simulink model "test_model"  (R2022b)
settings: Solver=VariableStepAuto  StartTime=0.0  StopTime=10.0  RelTol=1e-3
InitFcn:
  | parameters_test_model;
values from neighbouring files (symbols this model uses):
  A1 = [0.3, 0.3, 0.2]    [parameters_test_model.m]    (also in tensegrity_Val_like.m = [(G1+G2+G3)/3])
  a1 = 0.04    [parameters_test_model.m]
  b_all = 2*ones(6, 1)    [parameters_test_model.m]
  h1 = 0.5    [parameters_test_model.m]
  k_all = 1e3*ones(6, 1)    [parameters_test_model.m]
  l0_all = [l01, l02, l03, l04, l05, l06]'    [parameters_test_model.m]
  predpeti = 0.95    [parameters_test_model.m]
undefined symbols (not defined in the file or in its folder): X, Y, Z
libraries: sm_lib x21, nesl_utility x21
settings Model: Creator=zavrel  LastModifiedBy=zavrel
settings SolverCC: AlgebraicLoopSolver=TrustRegion
settings DebuggingCC: UnconnectedInputMsg=warning  UnconnectedOutputMsg=warning  UnconnectedLineMsg=warning  SFMachineParentedDataDiag=warning
settings ModelReferenceCC: EnableRefExpFcnMdlSchedulingChecks=on
settings RTWCC: DLArmComputeVersion=19.05

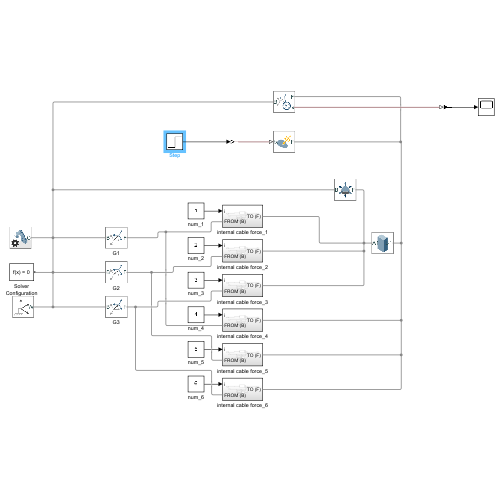
[thumbnail: Simulink's stored preview of the top-level diagram]
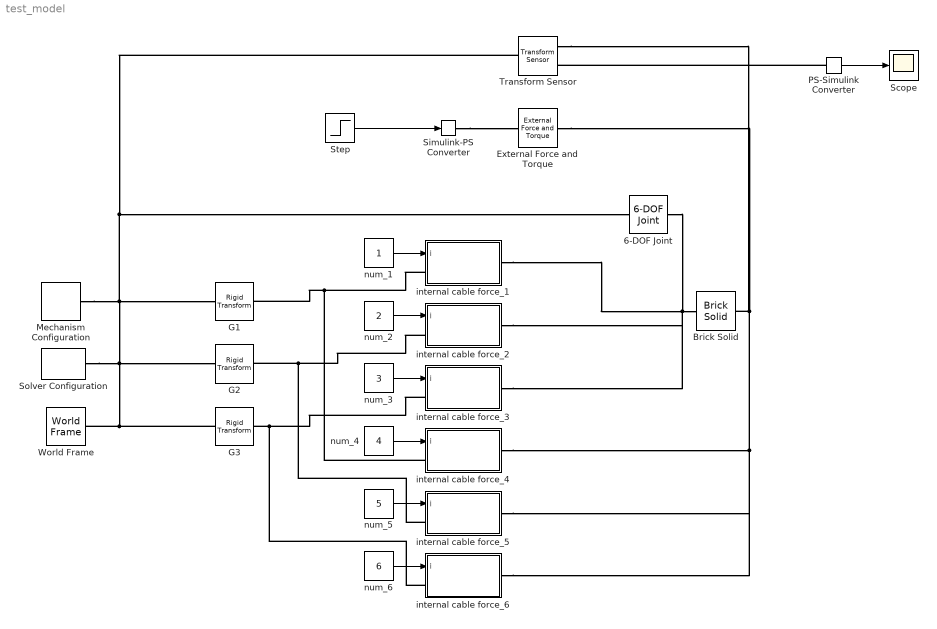
== system test_model ==
  6-DOF Joint : sm_lib/Joints/6-DOF Joint  JointMode=Normal  SenseConstraintForce=off  SenseConstraintForceX=off  SenseConstraintForceY=off  SenseConstraintForceZ=off  SenseConstraintTorque=off  SenseConstraintTorqueX=off  SenseConstraintTorqueY=off  SenseConstraintTorqueZ=off  SenseTotalForce=off  SenseTotalForceX=off  SenseTotalForceY=off  SenseTotalForceZ=off  SenseTotalTorque=off  SenseTotalTorqueX=off  SenseTotalTorqueY=off  SenseTotalTorqueZ=off  CompositeWrenchDir=FollowerOnBase  CompositeWrenchFrame=BaseFrame  PxEquilibriumPosition=0  PxEquilibriumPositionUnits=m  PxSpringStiffness=0  PxSpringStiffnessUnits=N/m  PxDampingCoefficient=0  PxDampingCoefficientUnits=N/(m/s)  PxTorqueActuationMode=NoTorque  PxMotionActuationMode=ComputedMotion  PxSensePosition=off  PxSenseVelocity=off  PxSenseAcceleration=off  PxSenseTorqueForce=off  PxSenseLowerLimitTorqueForce=off  PxSenseUpperLimitTorqueForce=off  PxLowerLimitSpecify=off  PxLowerLimitBound=-1  PxLowerLimitBoundUnits=m  PxLowerLimitStiffness=1e6  PxLowerLimitStiffnessUnits=N/m  PxLowerLimitDamping=1e3  PxLowerLimitDampingUnits=N/(m/s)  PxLowerLimitTransitionRegionWidth=1e-4  PxLowerLimitTransitionRegionWidthUnits=m  PxUpperLimitSpecify=off  PxUpperLimitBound=1  PxUpperLimitBoundUnits=m  PxUpperLimitStiffness=1e6  PxUpperLimitStiffnessUnits=N/m  PxUpperLimitDamping=1e3  PxUpperLimitDampingUnits=N/(m/s)  PxUpperLimitTransitionRegionWidth=1e-4  PxUpperLimitTransitionRegionWidthUnits=m  PxPositionTargetSpecify=on  PxPositionTargetPriority=Low  PxPositionTargetValue=A1(1)  PxPositionTargetValueUnits=m  PxVelocityTargetSpecify=off  PxVelocityTargetPriority=High  PxVelocityTargetValue=0  PxVelocityTargetValueUnits=m/s  PyEquilibriumPosition=0  PyEquilibriumPositionUnits=m  PySpringStiffness=0  PySpringStiffnessUnits=N/m  PyDampingCoefficient=0  PyDampingCoefficientUnits=N/(m/s)  PyTorqueActuationMode=NoTorque  PyMotionActuationMode=ComputedMotion  PySensePosition=off  PySenseVelocity=off  PySenseAcceleration=off  PySenseTorqueForce=off  PySenseLowerLimitTorqueForce=off  PySenseUpperLimitTorqueForce=off  PyLowerLimitSpecify=off  PyLowerLimitBound=-1  PyLowerLimitBoundUnits=m  PyLowerLimitStiffness=1e6  PyLowerLimitStiffnessUnits=N/m  PyLowerLimitDamping=1e3  PyLowerLimitDampingUnits=N/(m/s)  PyLowerLimitTransitionRegionWidth=1e-4  PyLowerLimitTransitionRegionWidthUnits=m  PyUpperLimitSpecify=off  PyUpperLimitBound=1  PyUpperLimitBoundUnits=m  PyUpperLimitStiffness=1e6  PyUpperLimitStiffnessUnits=N/m  PyUpperLimitDamping=1e3  PyUpperLimitDampingUnits=N/(m/s)  PyUpperLimitTransitionRegionWidth=1e-4  PyUpperLimitTransitionRegionWidthUnits=m  PyPositionTargetSpecify=on  PyPositionTargetPriority=Low  PyPositionTargetValue=A1(2)  PyPositionTargetValueUnits=m  PyVelocityTargetSpecify=off  PyVelocityTargetPriority=High  PyVelocityTargetValue=0  PyVelocityTargetValueUnits=m/s  PzEquilibriumPosition=0  PzEquilibriumPositionUnits=m  PzSpringStiffness=0  PzSpringStiffnessUnits=N/m  PzDampingCoefficient=0  PzDampingCoefficientUnits=N/(m/s)  PzTorqueActuationMode=NoTorque  PzMotionActuationMode=ComputedMotion  PzSensePosition=off  PzSenseVelocity=off  PzSenseAcceleration=off  PzSenseTorqueForce=off  PzSenseLowerLimitTorqueForce=off  PzSenseUpperLimitTorqueForce=off  PzLowerLimitSpecify=off  PzLowerLimitBound=-1  PzLowerLimitBoundUnits=m  PzLowerLimitStiffness=1e6  PzLowerLimitStiffnessUnits=N/m  PzLowerLimitDamping=1e3  PzLowerLimitDampingUnits=N/(m/s)  PzLowerLimitTransitionRegionWidth=1e-4  PzLowerLimitTransitionRegionWidthUnits=m  PzUpperLimitSpecify=off  PzUpperLimitBound=1  PzUpperLimitBoundUnits=m  PzUpperLimitStiffness=1e6  PzUpperLimitStiffnessUnits=N/m  PzUpperLimitDamping=1e3  PzUpperLimitDampingUnits=N/(m/s)  PzUpperLimitTransitionRegionWidth=1e-4  PzUpperLimitTransitionRegionWidthUnits=m  PzPositionTargetSpecify=on  PzPositionTargetPriority=Low  PzPositionTargetValue=A1(3)  PzPositionTargetValueUnits=m  PzVelocityTargetSpecify=off  PzVelocityTargetPriority=High  PzVelocityTargetValue=0  PzVelocityTargetValueUnits=m/s  SphEqPosRotationMethod=None  SphEqPosRotationAngleUnits=deg  SphEqPosRotationStandardAxis=+Z  SphEqPosRotationAngle=0.0  SphEqPosRotationArbitraryAxis=[0 0 1]  SphEqPosFollAlignAxisA=+X  SphEqPosBaseAlignAxisA=+Y  SphEqPosFollAlignAxisB=+Y  SphEqPosBaseAlignAxisB=+Z  SphEqPosRotationSequenceAxes=FollowerAxes  SphEqPosRotationSequence=XYX  SphEqPosRotationSequenceAngles=[0 0 0]  SphEqPosRotationSequenceAnglesUnits=deg  SphEqPosRotationMatrix=[1 0 0; 0 1 0; 0 0 1]  SphEqPosQuaternion=[1 0 0 0]  SphSpringStiffness=0  SphSpringStiffnessUnits=N*m/deg  SphDampingCoefficient=0  SphDampingCoefficientUnits=N*m/(deg/s)  SphActuateTorqueX=off  SphActuateTorqueY=off  SphActuateTorqueZ=off  SphActuateTorque=off  SphTorqueActuationMode=NoTorque  SphMotionActuationMode=ComputedMotion  SphActuationFrame=BaseFrame  SphSensePosition=off  SphSenseVelocityX=off  SphSenseVelocityY=off  SphSenseVelocityZ=off  SphSenseVelocity=off  SphSenseAccelerationX=off  SphSenseAccelerationY=off  SphSenseAccelerationZ=off  SphSenseAcceleration=off  SphSenseTorqueX=off  SphSenseTorqueY=off  SphSenseTorqueZ=off  SphSenseTorqueForce=off  SphSenseLowerLimitTorqueMag=off  SphSenseUpperLimitTorqueMag=off  SphSensingFrame=BaseFrame  SphLowerLimitSpecify=off  SphLowerLimitBound=15  SphLowerLimitBoundUnits=deg  SphLowerLimitStiffness=1e4  SphLowerLimitStiffnessUnits=N*m/deg  SphLowerLimitDamping=10  SphLowerLimitDampingUnits=N*m/(deg/s)  SphLowerLimitTransitionRegionWidth=0.1  SphLowerLimitTransitionRegionWidthUnits=deg  SphUpperLimitSpecify=off  SphUpperLimitBound=45  SphUpperLimitBoundUnits=deg  SphUpperLimitStiffness=1e4  SphUpperLimitStiffnessUnits=N*m/deg  SphUpperLimitDamping=10  SphUpperLimitDampingUnits=N*m/(deg/s)  SphUpperLimitTransitionRegionWidth=0.1  SphUpperLimitTransitionRegionWidthUnits=deg  SphPositionTargetRotationMethod=RotationSequence  SphPositionTargetRotationAngleUnits=deg  SphPositionTargetRotationStandardAxis=+Z  SphPositionTargetRotationAngle=0.0  SphPositionTargetRotationArbitraryAxis=[0 0 1]  SphPositionTargetFollAlignAxisA=+X  SphPositionTargetBaseAlignAxisA=+Y  SphPositionTargetFollAlignAxisB=+Y  SphPositionTargetBaseAlignAxisB=+Z  SphPositionTargetRotationSequenceAxes=FollowerAxes  SphPositionTargetRotationSequence=XYZ  SphPositionTargetRotationSequenceAngles=[0 0 0]  SphPositionTargetRotationSequenceAnglesUnits=deg  SphPositionTargetRotationMatrix=[1 0 0; 0 1 0; 0 0 1]  SphPositionTargetQuaternion=[1 0 0 0]  SphPositionTargetSpecify=on  SphPositionTargetPriority=Low  SphVelocityTargetValue=[0 0 0]  SphVelocityTargetValueUnits=deg/s  SphVelocityTargetSpecify=off  SphVelocityTargetPriority=High  SphVelocityTargetInFollowerFrame=on
  Brick Solid : sm_lib/Body Elements/Brick Solid  GraphicAmbientColor=[0.15 0.15 0.15 1.0]  BasedOnType=Density  BrickDimensions=[a1 a1 h1]  BrickDimensionUnits=m  CenterOfMass=[0 0 0]  CenterOfMassUnits=m  GraphicDiffuseColor=[0.5 0.5 0.5]  Density=1000  DensityUnits=kg/m^3  DoExposeReferenceFrame=off  GraphicEmissiveColor=[0.0 0.0 0.0 1.0]  ExportEntireGeometry=off  SerializedFrames=<Frames><Frame><Id>Frame1</Id><Value><Name>A1</Name><Origin><Source>GeometricFeature</Source><FeatureName>-z surface</FeatureName></Origin><PrimaryAxis><DefinedDirection>+Z</DefinedDirection><Source>ReferenceFrame</Source><SourceDirection>+Z</SourceDirection><FeatureName></FeatureName></PrimaryAxis><SecondaryAxis><DefinedDirection>+X</DefinedDirection><Source>ReferenceFrame</Source><SourceDirection>+X</SourceDirection><FeatureName></FeatureName></SecondaryAxis></Value></Frame><Frame><Id>Frame2</Id><Value><Name>B1</Name><Origin><Source>GeometricFeature</Source><FeatureName>+z surface</FeatureName></Origin><PrimaryAxis><DefinedDirection>+Z</DefinedDirection><Source>ReferenceFrame</Source><SourceDirection>+Z</SourceDirection><FeatureName></FeatureName></PrimaryAxis><SecondaryAxis><DefinedDirection>+X</DefinedDirection><Source>ReferenceFrame</Source><SourceDirection>+X</SourceDirection><FeatureName></FeatureName></SecondaryAxis></Value></Frame></Frames>  MarkerShape=Sphere  MarkerSize=10  GraphicType=FromGeometry  InertiaType=CalculateFromGeometry  Mass=1  MassUnits=kg  MomentsOfInertia=[1 1 1]  MomentsOfInertiaUnits=kg*m^2  GraphicOpacity=1.0  ProductsOfInertia=[0 0 0]  ProductsOfInertiaUnits=kg*m^2  GraphicShininess=75  GraphicSpecularColor=[0.5 0.5 0.5 1.0]  GraphicVisPropType=SimpleVisualProperties
  External Force and Torque : sm_lib/Forces and Torques/External Force and Torque  ForceResolutionFrame=World  EnableForceX=on  EnableForceY=off  EnableForceZ=off  EnableForce=off  TorqueResolutionFrame=AttachedFrame  EnableTorqueX=off  EnableTorqueY=off  EnableTorqueZ=off  EnableTorque=off
  G1 : sm_lib/Frames and Transforms/Rigid Transform  TranslationMethod=Cartesian  TranslationStandardOffset=0  TranslationLengthUnit=m  TranslationStandardAxis=+Z  TranslationCartesianOffset=G1  TranslationROffset=0  TranslationROffsetUnits=m  TranslationZOffset=0  TranslationZOffsetUnits=m  TranslationThetaOffset=0  TranslationThetaOffsetUnits=deg  RotationMethod=None  RotationAngleUnits=deg  RotationStandardAxis=+Z  RotationAngle=0.0  RotationArbitraryAxis=[0 0 1]  FollAlignAxisA=+X  BaseAlignAxisA=+Y  FollAlignAxisB=+Y  BaseAlignAxisB=+Z  RotationSequenceAxes=FollowerAxes  RotationSequence=XYX  RotationSequenceAngles=[0 0 0]  RotationSequenceAnglesUnits=deg  RotationMatrix=[1 0 0; 0 1 0; 0 0 1]  Quaternion=[1 0 0 0]
  G2 : sm_lib/Frames and Transforms/Rigid Transform  TranslationMethod=Cartesian  TranslationStandardOffset=0  TranslationLengthUnit=m  TranslationStandardAxis=+Z  TranslationCartesianOffset=G2  TranslationROffset=0  TranslationROffsetUnits=m  TranslationZOffset=0  TranslationZOffsetUnits=m  TranslationThetaOffset=0  TranslationThetaOffsetUnits=deg  RotationMethod=None  RotationAngleUnits=deg  RotationStandardAxis=+Z  RotationAngle=0.0  RotationArbitraryAxis=[0 0 1]  FollAlignAxisA=+X  BaseAlignAxisA=+Y  FollAlignAxisB=+Y  BaseAlignAxisB=+Z  RotationSequenceAxes=FollowerAxes  RotationSequence=XYX  RotationSequenceAngles=[0 0 0]  RotationSequenceAnglesUnits=deg  RotationMatrix=[1 0 0; 0 1 0; 0 0 1]  Quaternion=[1 0 0 0]
  G3 : sm_lib/Frames and Transforms/Rigid Transform  TranslationMethod=Cartesian  TranslationStandardOffset=0  TranslationLengthUnit=m  TranslationStandardAxis=+Z  TranslationCartesianOffset=G3  TranslationROffset=0  TranslationROffsetUnits=m  TranslationZOffset=0  TranslationZOffsetUnits=m  TranslationThetaOffset=0  TranslationThetaOffsetUnits=deg  RotationMethod=None  RotationAngleUnits=deg  RotationStandardAxis=+Z  RotationAngle=0.0  RotationArbitraryAxis=[0 0 1]  FollAlignAxisA=+X  BaseAlignAxisA=+Y  FollAlignAxisB=+Y  BaseAlignAxisB=+Z  RotationSequenceAxes=FollowerAxes  RotationSequence=XYX  RotationSequenceAngles=[0 0 0]  RotationSequenceAnglesUnits=deg  RotationMatrix=[1 0 0; 0 1 0; 0 0 1]  Quaternion=[1 0 0 0]
  Mechanism Configuration : sm_lib/Utilities/Mechanism Configuration  UniformGravity=Constant  GravityVector=[0 0 -9.80665]  GravityUnits=m/s^2  LinearizationDelta=0.001  JointModeTransitionNonlinearIterations=2
  PS-Simulink Converter : nesl_utility/PS-Simulink Converter  PhysicalDomain=network_engine_domain  SubClassName=ps_output  LeftPortType=input  RightPortType=output  PseudoPeriodic=off  Frequencies=[]  VectorFormat=inherit  Unit=inherit  AffineConversion=off
  Scope : Scope
  Simulink-PS Converter : nesl_utility/Simulink-PS Converter  PhysicalDomain=network_engine_domain  SubClassName=ps_input  LeftPortType=input  RightPortType=output  PseudoPeriodic=off  Frequencies=[]  NoiseDistribution=none  NoiseParameters=[]  Unit=1  AffineConversion=off  FilteringAndDerivatives=provide  SimscapeFilterOrder=1  InputFilterTimeConstant=0.001  UdotUserProvided=0
  Solver Configuration : nesl_utility/Solver Configuration  PhysicalDomain=network_engine_domain  SubClassName=solver  LeftPortType=input  RightPortType=generic  Tones=[]  Harmonics=[]  SimulateNoise=off  Profile=off  UseLocalSampling=off  EnableSwitchedLinearOptims=on  FrequencyDomain=off  UseCCode=off  RelTol=0.001  AbsTol=1e-06  MinStep=1e-09  ToWorkspace=off  RevertToSquareIcSolve=off  NumHomotopyIterations=100  PhasorMode=off  PhasorModeNumHarmonics=1  ConsistencySolver=NEWTON_FTOL  IndexReductionMethod=DerivativeReplacement  DoDC=off  ResidualTolerance=1e-09  ConsistencyTolSource=GLOBAL  ConsistencyAbsTol=0.001  ConsistencyRelTol=0.001  ConsistencyTolFactor=0.001  UseLocalSolver=off  LocalSolverChoice=NE_BACKWARD_EULER_ADVANCER  ResolveIndetEquations=on  FunctionEvalNumThread=1  LocalSolverSampleTime=0.001  DoFixedCost=off  MaxNonlinIter=3  MaxModeIter=2  ComputeImpulses=off  ImpulseIterations=2  LinearAlgebra=auto  LinearAlgebraNumThread=0  EquationFormulation=NE_TIME_EF  DelaysMemoryBudget=1024  AutomaticFiltering=on  FilteringTimeConstant=0.001  PartitionStorageMethod=AS_NEEDED  PartitionMemoryBudget=1024  PartitionMethod=ROBUST
  Step : Step  Time=5  After=100  SampleTime=0
  Transform Sensor : sm_lib/Frames and Transforms/Transform Sensor  MeasurementFrame=World  SenseAngle=off  SenseAxis=off  SenseQ=off  SenseR=off  SenseRotationSequence=off  RotationSequence=XYX  SenseOmegaX=off  SenseOmegaY=off  SenseOmegaZ=off  SenseQDot=off  SenseRDot=off  SenseAlphaX=off  SenseAlphaY=off  SenseAlphaZ=off  SenseQDDot=off  SenseRDDot=off  SenseX=on  SenseY=off  SenseZ=off  SenseRad=off  SenseAzim=off  SenseDist=off  SenseInc=off  SenseXDot=off  SenseYDot=off  SenseZDot=off  SenseRadDot=off  SenseAzimDot=off  SenseDistDot=off  SenseIncDot=off  SenseXDDot=off  SenseYDDot=off  SenseZDDot=off  SenseRadDDot=off  SenseAzimDDot=off  SenseDistDDot=off  SenseIncDDot=off
  World Frame : sm_lib/Frames and Transforms/World Frame
  internal cable force_1 : Subsystem
  internal cable force_2 : Subsystem
  internal cable force_3 : Subsystem
  internal cable force_4 : Subsystem
  internal cable force_5 : Subsystem
  internal cable force_6 : Subsystem
  num_1 : Constant
  num_2 : Constant  Value=2
  num_3 : Constant  Value=3
  num_4 : Constant  Value=4
  num_5 : Constant  Value=5
  num_6 : Constant  Value=6
  wires:
  num_1/1 -> internal cable force_1/1(i)
  num_2/1 -> internal cable force_2/1(i)
  num_3/1 -> internal cable force_3/1(i)
  num_4/1 -> internal cable force_4/1(i)
  num_5/1 -> internal cable force_5/1(i)
  num_6/1 -> internal cable force_6/1(i)
  Step/1 -> Simulink-PS Converter/1
  PS-Simulink Converter/1 -> Scope/1
  connections:
  Mechanism Configuration/RConn1 -- Transform Sensor/LConn1 -- 6-DOF Joint/LConn1 -- Solver Configuration/RConn1 -- G2/LConn1 -- G3/LConn1 -- World Frame/RConn1 -- G1/LConn1
  internal cable force_1/LConn1 -- internal cable force_4/LConn1 -- G1/RConn1
  internal cable force_2/LConn1 -- internal cable force_5/LConn1 -- G2/RConn1
  internal cable force_3/LConn1 -- internal cable force_6/LConn1 -- G3/RConn1
  internal cable force_1/RConn1 -- 6-DOF Joint/RConn1 -- internal cable force_3/RConn1 -- internal cable force_2/RConn1 -- Brick Solid/LConn1
  internal cable force_4/RConn1 -- internal cable force_6/RConn1 -- internal cable force_5/RConn1 -- Transform Sensor/RConn1 -- External Force and Torque/RConn1 -- Brick Solid/RConn1
  Simulink-PS Converter/RConn1 -- External Force and Torque/LConn1
  PS-Simulink Converter/LConn1 -- Transform Sensor/RConn2

== system test_model/internal cable force_1 ==
  i : Inport
  Gain : Gain  Gain=-1
  Internal Force : sm_lib/Forces and Torques/Internal Force
  Simulink-PS Converter : nesl_utility/Simulink-PS Converter  PhysicalDomain=network_engine_domain  SubClassName=ps_input  LeftPortType=input  RightPortType=output  PseudoPeriodic=off  Frequencies=[]  NoiseDistribution=none  NoiseParameters=[]  Unit=1  AffineConversion=off  FilteringAndDerivatives=provide  SimscapeFilterOrder=1  InputFilterTimeConstant=0.001  UdotUserProvided=0
  cable force : Subsystem
  TO (F) : PMIOPort  Side=Right
  FROM (B) : PMIOPort  Port=2  Side=Left
  wires:
  cable force/1(Fc) -> Gain/1
  Gain/1 -> Simulink-PS Converter/1
  i/1 -> cable force/1(i)
  connections:
  Simulink-PS Converter/RConn1 -- Internal Force/LConn2
  cable force/RConn1 -- TO (F)/RConn1 -- Internal Force/RConn1
  cable force/RConn2 -- Internal Force/LConn1 -- FROM (B)/RConn1

== system test_model/internal cable force_2 ==
  i : Inport
  Gain : Gain  Gain=-1
  Internal Force : sm_lib/Forces and Torques/Internal Force
  Simulink-PS Converter : nesl_utility/Simulink-PS Converter  PhysicalDomain=network_engine_domain  SubClassName=ps_input  LeftPortType=input  RightPortType=output  PseudoPeriodic=off  Frequencies=[]  NoiseDistribution=none  NoiseParameters=[]  Unit=1  AffineConversion=off  FilteringAndDerivatives=provide  SimscapeFilterOrder=1  InputFilterTimeConstant=0.001  UdotUserProvided=0
  cable force : Subsystem
  TO (F) : PMIOPort  Side=Right
  FROM (B) : PMIOPort  Port=2  Side=Left
  wires:
  i/1 -> cable force/1(i)
  Gain/1 -> Simulink-PS Converter/1
  cable force/1(Fc) -> Gain/1
  connections:
  FROM (B)/RConn1 -- Internal Force/LConn1 -- cable force/RConn2
  Internal Force/RConn1 -- TO (F)/RConn1 -- cable force/RConn1
  Simulink-PS Converter/RConn1 -- Internal Force/LConn2

== system test_model/internal cable force_3 ==
  i : Inport
  Gain : Gain  Gain=-1
  Internal Force : sm_lib/Forces and Torques/Internal Force
  Simulink-PS Converter : nesl_utility/Simulink-PS Converter  PhysicalDomain=network_engine_domain  SubClassName=ps_input  LeftPortType=input  RightPortType=output  PseudoPeriodic=off  Frequencies=[]  NoiseDistribution=none  NoiseParameters=[]  Unit=1  AffineConversion=off  FilteringAndDerivatives=provide  SimscapeFilterOrder=1  InputFilterTimeConstant=0.001  UdotUserProvided=0
  cable force : Subsystem
  TO (F) : PMIOPort  Side=Right
  FROM (B) : PMIOPort  Port=2  Side=Left
  wires:
  cable force/1(Fc) -> Gain/1
  Gain/1 -> Simulink-PS Converter/1
  i/1 -> cable force/1(i)
  connections:
  Simulink-PS Converter/RConn1 -- Internal Force/LConn2
  cable force/RConn1 -- TO (F)/RConn1 -- Internal Force/RConn1
  cable force/RConn2 -- Internal Force/LConn1 -- FROM (B)/RConn1

== system test_model/internal cable force_4 ==
  i : Inport
  Gain : Gain  Gain=-1
  Internal Force : sm_lib/Forces and Torques/Internal Force
  Simulink-PS Converter : nesl_utility/Simulink-PS Converter  PhysicalDomain=network_engine_domain  SubClassName=ps_input  LeftPortType=input  RightPortType=output  PseudoPeriodic=off  Frequencies=[]  NoiseDistribution=none  NoiseParameters=[]  Unit=1  AffineConversion=off  FilteringAndDerivatives=provide  SimscapeFilterOrder=1  InputFilterTimeConstant=0.001  UdotUserProvided=0
  cable force : Subsystem
  TO (F) : PMIOPort  Side=Right
  FROM (B) : PMIOPort  Port=2  Side=Left
  wires:
  i/1 -> cable force/1(i)
  Gain/1 -> Simulink-PS Converter/1
  cable force/1(Fc) -> Gain/1
  connections:
  FROM (B)/RConn1 -- Internal Force/LConn1 -- cable force/RConn2
  Internal Force/RConn1 -- TO (F)/RConn1 -- cable force/RConn1
  Simulink-PS Converter/RConn1 -- Internal Force/LConn2

== system test_model/internal cable force_5 ==
  i : Inport
  Gain : Gain  Gain=-1
  Internal Force : sm_lib/Forces and Torques/Internal Force
  Simulink-PS Converter : nesl_utility/Simulink-PS Converter  PhysicalDomain=network_engine_domain  SubClassName=ps_input  LeftPortType=input  RightPortType=output  PseudoPeriodic=off  Frequencies=[]  NoiseDistribution=none  NoiseParameters=[]  Unit=1  AffineConversion=off  FilteringAndDerivatives=provide  SimscapeFilterOrder=1  InputFilterTimeConstant=0.001  UdotUserProvided=0
  cable force : Subsystem
  TO (F) : PMIOPort  Side=Right
  FROM (B) : PMIOPort  Port=2  Side=Left
  wires:
  cable force/1(Fc) -> Gain/1
  Gain/1 -> Simulink-PS Converter/1
  i/1 -> cable force/1(i)
  connections:
  Simulink-PS Converter/RConn1 -- Internal Force/LConn2
  cable force/RConn1 -- TO (F)/RConn1 -- Internal Force/RConn1
  cable force/RConn2 -- Internal Force/LConn1 -- FROM (B)/RConn1

== system test_model/internal cable force_6 ==
  i : Inport
  Gain : Gain  Gain=-1
  Internal Force : sm_lib/Forces and Torques/Internal Force
  Simulink-PS Converter : nesl_utility/Simulink-PS Converter  PhysicalDomain=network_engine_domain  SubClassName=ps_input  LeftPortType=input  RightPortType=output  PseudoPeriodic=off  Frequencies=[]  NoiseDistribution=none  NoiseParameters=[]  Unit=1  AffineConversion=off  FilteringAndDerivatives=provide  SimscapeFilterOrder=1  InputFilterTimeConstant=0.001  UdotUserProvided=0
  cable force : Subsystem
  TO (F) : PMIOPort  Side=Right
  FROM (B) : PMIOPort  Port=2  Side=Left
  wires:
  i/1 -> cable force/1(i)
  Gain/1 -> Simulink-PS Converter/1
  cable force/1(Fc) -> Gain/1
  connections:
  FROM (B)/RConn1 -- Internal Force/LConn1 -- cable force/RConn2
  Internal Force/RConn1 -- TO (F)/RConn1 -- cable force/RConn1
  Simulink-PS Converter/RConn1 -- Internal Force/LConn2

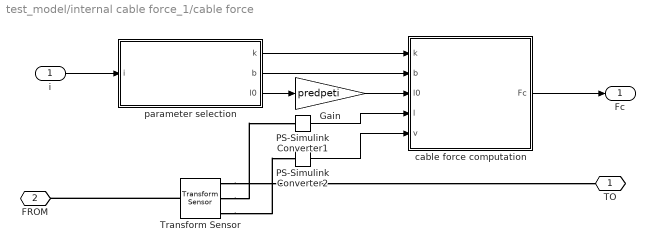
== system test_model/internal cable force_1/cable force ==
  i : Inport
  Gain : Gain  Gain=predpeti
  PS-Simulink Converter1 : nesl_utility/PS-Simulink Converter  PhysicalDomain=network_engine_domain  SubClassName=ps_output  LeftPortType=input  RightPortType=output  PseudoPeriodic=off  Frequencies=[]  VectorFormat=1-D array  Unit=inherit  AffineConversion=off
  PS-Simulink Converter2 : nesl_utility/PS-Simulink Converter  PhysicalDomain=network_engine_domain  SubClassName=ps_output  LeftPortType=input  RightPortType=output  PseudoPeriodic=off  Frequencies=[]  VectorFormat=1-D array  Unit=inherit  AffineConversion=off
  Transform Sensor : sm_lib/Frames and Transforms/Transform Sensor  MeasurementFrame=World  SenseAngle=off  SenseAxis=off  SenseQ=off  SenseR=off  SenseRotationSequence=off  RotationSequence=XYX  SenseOmegaX=off  SenseOmegaY=off  SenseOmegaZ=off  SenseQDot=off  SenseRDot=off  SenseAlphaX=off  SenseAlphaY=off  SenseAlphaZ=off  SenseQDDot=off  SenseRDDot=off  SenseX=off  SenseY=off  SenseZ=off  SenseRad=off  SenseAzim=off  SenseDist=on  SenseInc=off  SenseXDot=off  SenseYDot=off  SenseZDot=off  SenseRadDot=off  SenseAzimDot=off  SenseDistDot=on  SenseIncDot=off  SenseXDDot=off  SenseYDDot=off  SenseZDDot=off  SenseRadDDot=off  SenseAzimDDot=off  SenseDistDDot=off  SenseIncDDot=off
  cable force computation : MATLAB Function  TreatAsAtomicUnit=on
  parameter selection : Subsystem
  TO : PMIOPort  Side=Right
  FROM : PMIOPort  Port=2  Side=Right
  Fc : Outport
  wires:
  Gain/1 -> cable force computation/3(l0)
  cable force computation/1(Fc) -> Fc/1
  parameter selection/2(b) -> cable force computation/2(b)
  parameter selection/3(l0) -> Gain/1
  parameter selection/1(k) -> cable force computation/1(k)
  PS-Simulink Converter1/1 -> cable force computation/4(l)
  PS-Simulink Converter2/1 -> cable force computation/5(v)
  i/1 -> parameter selection/1(i)
  connections:
  Transform Sensor/RConn3 -- PS-Simulink Converter2/LConn1
  Transform Sensor/RConn2 -- PS-Simulink Converter1/LConn1
  Transform Sensor/RConn1 -- TO/RConn1
  Transform Sensor/LConn1 -- FROM/RConn1

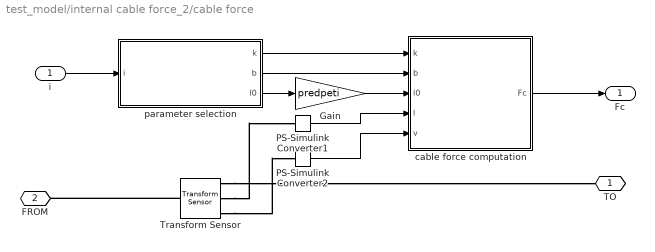
== system test_model/internal cable force_2/cable force ==
  i : Inport
  Gain : Gain  Gain=predpeti
  PS-Simulink Converter1 : nesl_utility/PS-Simulink Converter  PhysicalDomain=network_engine_domain  SubClassName=ps_output  LeftPortType=input  RightPortType=output  PseudoPeriodic=off  Frequencies=[]  VectorFormat=1-D array  Unit=inherit  AffineConversion=off
  PS-Simulink Converter2 : nesl_utility/PS-Simulink Converter  PhysicalDomain=network_engine_domain  SubClassName=ps_output  LeftPortType=input  RightPortType=output  PseudoPeriodic=off  Frequencies=[]  VectorFormat=1-D array  Unit=inherit  AffineConversion=off
  Transform Sensor : sm_lib/Frames and Transforms/Transform Sensor  MeasurementFrame=World  SenseAngle=off  SenseAxis=off  SenseQ=off  SenseR=off  SenseRotationSequence=off  RotationSequence=XYX  SenseOmegaX=off  SenseOmegaY=off  SenseOmegaZ=off  SenseQDot=off  SenseRDot=off  SenseAlphaX=off  SenseAlphaY=off  SenseAlphaZ=off  SenseQDDot=off  SenseRDDot=off  SenseX=off  SenseY=off  SenseZ=off  SenseRad=off  SenseAzim=off  SenseDist=on  SenseInc=off  SenseXDot=off  SenseYDot=off  SenseZDot=off  SenseRadDot=off  SenseAzimDot=off  SenseDistDot=on  SenseIncDot=off  SenseXDDot=off  SenseYDDot=off  SenseZDDot=off  SenseRadDDot=off  SenseAzimDDot=off  SenseDistDDot=off  SenseIncDDot=off
  cable force computation : MATLAB Function  TreatAsAtomicUnit=on
  parameter selection : Subsystem
  TO : PMIOPort  Side=Right
  FROM : PMIOPort  Port=2  Side=Right
  Fc : Outport
  wires:
  i/1 -> parameter selection/1(i)
  PS-Simulink Converter2/1 -> cable force computation/5(v)
  PS-Simulink Converter1/1 -> cable force computation/4(l)
  parameter selection/1(k) -> cable force computation/1(k)
  parameter selection/3(l0) -> Gain/1
  parameter selection/2(b) -> cable force computation/2(b)
  cable force computation/1(Fc) -> Fc/1
  Gain/1 -> cable force computation/3(l0)
  connections:
  Transform Sensor/LConn1 -- FROM/RConn1
  Transform Sensor/RConn1 -- TO/RConn1
  Transform Sensor/RConn2 -- PS-Simulink Converter1/LConn1
  Transform Sensor/RConn3 -- PS-Simulink Converter2/LConn1

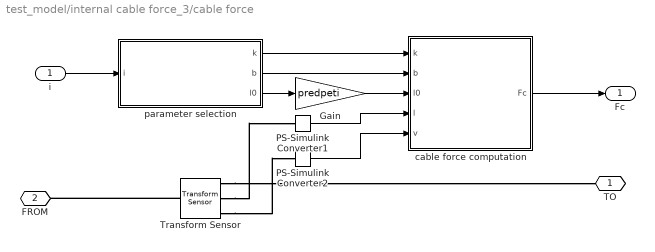
== system test_model/internal cable force_3/cable force ==
  i : Inport
  Gain : Gain  Gain=predpeti
  PS-Simulink Converter1 : nesl_utility/PS-Simulink Converter  PhysicalDomain=network_engine_domain  SubClassName=ps_output  LeftPortType=input  RightPortType=output  PseudoPeriodic=off  Frequencies=[]  VectorFormat=1-D array  Unit=inherit  AffineConversion=off
  PS-Simulink Converter2 : nesl_utility/PS-Simulink Converter  PhysicalDomain=network_engine_domain  SubClassName=ps_output  LeftPortType=input  RightPortType=output  PseudoPeriodic=off  Frequencies=[]  VectorFormat=1-D array  Unit=inherit  AffineConversion=off
  Transform Sensor : sm_lib/Frames and Transforms/Transform Sensor  MeasurementFrame=World  SenseAngle=off  SenseAxis=off  SenseQ=off  SenseR=off  SenseRotationSequence=off  RotationSequence=XYX  SenseOmegaX=off  SenseOmegaY=off  SenseOmegaZ=off  SenseQDot=off  SenseRDot=off  SenseAlphaX=off  SenseAlphaY=off  SenseAlphaZ=off  SenseQDDot=off  SenseRDDot=off  SenseX=off  SenseY=off  SenseZ=off  SenseRad=off  SenseAzim=off  SenseDist=on  SenseInc=off  SenseXDot=off  SenseYDot=off  SenseZDot=off  SenseRadDot=off  SenseAzimDot=off  SenseDistDot=on  SenseIncDot=off  SenseXDDot=off  SenseYDDot=off  SenseZDDot=off  SenseRadDDot=off  SenseAzimDDot=off  SenseDistDDot=off  SenseIncDDot=off
  cable force computation : MATLAB Function  TreatAsAtomicUnit=on
  parameter selection : Subsystem
  TO : PMIOPort  Side=Right
  FROM : PMIOPort  Port=2  Side=Right
  Fc : Outport
  wires:
  Gain/1 -> cable force computation/3(l0)
  cable force computation/1(Fc) -> Fc/1
  parameter selection/2(b) -> cable force computation/2(b)
  parameter selection/3(l0) -> Gain/1
  parameter selection/1(k) -> cable force computation/1(k)
  PS-Simulink Converter1/1 -> cable force computation/4(l)
  PS-Simulink Converter2/1 -> cable force computation/5(v)
  i/1 -> parameter selection/1(i)
  connections:
  Transform Sensor/RConn3 -- PS-Simulink Converter2/LConn1
  Transform Sensor/RConn2 -- PS-Simulink Converter1/LConn1
  Transform Sensor/RConn1 -- TO/RConn1
  Transform Sensor/LConn1 -- FROM/RConn1

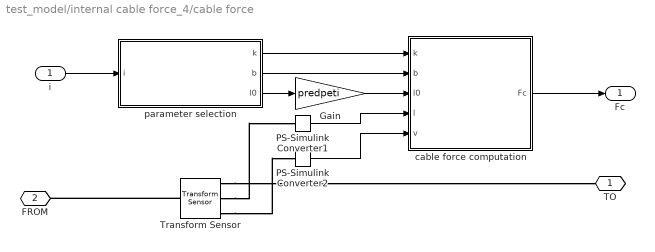
== system test_model/internal cable force_4/cable force ==
  i : Inport
  Gain : Gain  Gain=predpeti
  PS-Simulink Converter1 : nesl_utility/PS-Simulink Converter  PhysicalDomain=network_engine_domain  SubClassName=ps_output  LeftPortType=input  RightPortType=output  PseudoPeriodic=off  Frequencies=[]  VectorFormat=1-D array  Unit=inherit  AffineConversion=off
  PS-Simulink Converter2 : nesl_utility/PS-Simulink Converter  PhysicalDomain=network_engine_domain  SubClassName=ps_output  LeftPortType=input  RightPortType=output  PseudoPeriodic=off  Frequencies=[]  VectorFormat=1-D array  Unit=inherit  AffineConversion=off
  Transform Sensor : sm_lib/Frames and Transforms/Transform Sensor  MeasurementFrame=World  SenseAngle=off  SenseAxis=off  SenseQ=off  SenseR=off  SenseRotationSequence=off  RotationSequence=XYX  SenseOmegaX=off  SenseOmegaY=off  SenseOmegaZ=off  SenseQDot=off  SenseRDot=off  SenseAlphaX=off  SenseAlphaY=off  SenseAlphaZ=off  SenseQDDot=off  SenseRDDot=off  SenseX=off  SenseY=off  SenseZ=off  SenseRad=off  SenseAzim=off  SenseDist=on  SenseInc=off  SenseXDot=off  SenseYDot=off  SenseZDot=off  SenseRadDot=off  SenseAzimDot=off  SenseDistDot=on  SenseIncDot=off  SenseXDDot=off  SenseYDDot=off  SenseZDDot=off  SenseRadDDot=off  SenseAzimDDot=off  SenseDistDDot=off  SenseIncDDot=off
  cable force computation : MATLAB Function  TreatAsAtomicUnit=on
  parameter selection : Subsystem
  TO : PMIOPort  Side=Right
  FROM : PMIOPort  Port=2  Side=Right
  Fc : Outport
  wires:
  i/1 -> parameter selection/1(i)
  PS-Simulink Converter2/1 -> cable force computation/5(v)
  PS-Simulink Converter1/1 -> cable force computation/4(l)
  parameter selection/1(k) -> cable force computation/1(k)
  parameter selection/3(l0) -> Gain/1
  parameter selection/2(b) -> cable force computation/2(b)
  cable force computation/1(Fc) -> Fc/1
  Gain/1 -> cable force computation/3(l0)
  connections:
  Transform Sensor/LConn1 -- FROM/RConn1
  Transform Sensor/RConn1 -- TO/RConn1
  Transform Sensor/RConn2 -- PS-Simulink Converter1/LConn1
  Transform Sensor/RConn3 -- PS-Simulink Converter2/LConn1

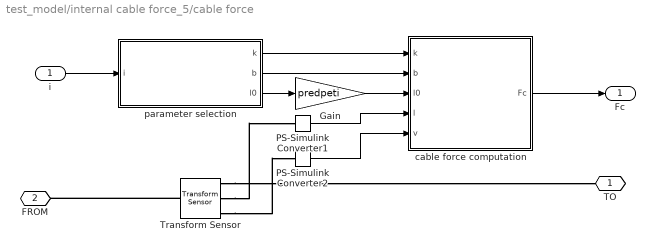
== system test_model/internal cable force_5/cable force ==
  i : Inport
  Gain : Gain  Gain=predpeti
  PS-Simulink Converter1 : nesl_utility/PS-Simulink Converter  PhysicalDomain=network_engine_domain  SubClassName=ps_output  LeftPortType=input  RightPortType=output  PseudoPeriodic=off  Frequencies=[]  VectorFormat=1-D array  Unit=inherit  AffineConversion=off
  PS-Simulink Converter2 : nesl_utility/PS-Simulink Converter  PhysicalDomain=network_engine_domain  SubClassName=ps_output  LeftPortType=input  RightPortType=output  PseudoPeriodic=off  Frequencies=[]  VectorFormat=1-D array  Unit=inherit  AffineConversion=off
  Transform Sensor : sm_lib/Frames and Transforms/Transform Sensor  MeasurementFrame=World  SenseAngle=off  SenseAxis=off  SenseQ=off  SenseR=off  SenseRotationSequence=off  RotationSequence=XYX  SenseOmegaX=off  SenseOmegaY=off  SenseOmegaZ=off  SenseQDot=off  SenseRDot=off  SenseAlphaX=off  SenseAlphaY=off  SenseAlphaZ=off  SenseQDDot=off  SenseRDDot=off  SenseX=off  SenseY=off  SenseZ=off  SenseRad=off  SenseAzim=off  SenseDist=on  SenseInc=off  SenseXDot=off  SenseYDot=off  SenseZDot=off  SenseRadDot=off  SenseAzimDot=off  SenseDistDot=on  SenseIncDot=off  SenseXDDot=off  SenseYDDot=off  SenseZDDot=off  SenseRadDDot=off  SenseAzimDDot=off  SenseDistDDot=off  SenseIncDDot=off
  cable force computation : MATLAB Function  TreatAsAtomicUnit=on
  parameter selection : Subsystem
  TO : PMIOPort  Side=Right
  FROM : PMIOPort  Port=2  Side=Right
  Fc : Outport
  wires:
  Gain/1 -> cable force computation/3(l0)
  cable force computation/1(Fc) -> Fc/1
  parameter selection/2(b) -> cable force computation/2(b)
  parameter selection/3(l0) -> Gain/1
  parameter selection/1(k) -> cable force computation/1(k)
  PS-Simulink Converter1/1 -> cable force computation/4(l)
  PS-Simulink Converter2/1 -> cable force computation/5(v)
  i/1 -> parameter selection/1(i)
  connections:
  Transform Sensor/RConn3 -- PS-Simulink Converter2/LConn1
  Transform Sensor/RConn2 -- PS-Simulink Converter1/LConn1
  Transform Sensor/RConn1 -- TO/RConn1
  Transform Sensor/LConn1 -- FROM/RConn1

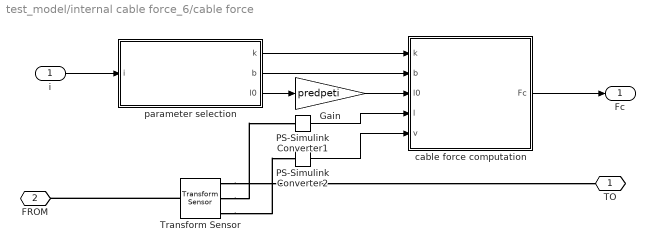
== system test_model/internal cable force_6/cable force ==
  i : Inport
  Gain : Gain  Gain=predpeti
  PS-Simulink Converter1 : nesl_utility/PS-Simulink Converter  PhysicalDomain=network_engine_domain  SubClassName=ps_output  LeftPortType=input  RightPortType=output  PseudoPeriodic=off  Frequencies=[]  VectorFormat=1-D array  Unit=inherit  AffineConversion=off
  PS-Simulink Converter2 : nesl_utility/PS-Simulink Converter  PhysicalDomain=network_engine_domain  SubClassName=ps_output  LeftPortType=input  RightPortType=output  PseudoPeriodic=off  Frequencies=[]  VectorFormat=1-D array  Unit=inherit  AffineConversion=off
  Transform Sensor : sm_lib/Frames and Transforms/Transform Sensor  MeasurementFrame=World  SenseAngle=off  SenseAxis=off  SenseQ=off  SenseR=off  SenseRotationSequence=off  RotationSequence=XYX  SenseOmegaX=off  SenseOmegaY=off  SenseOmegaZ=off  SenseQDot=off  SenseRDot=off  SenseAlphaX=off  SenseAlphaY=off  SenseAlphaZ=off  SenseQDDot=off  SenseRDDot=off  SenseX=off  SenseY=off  SenseZ=off  SenseRad=off  SenseAzim=off  SenseDist=on  SenseInc=off  SenseXDot=off  SenseYDot=off  SenseZDot=off  SenseRadDot=off  SenseAzimDot=off  SenseDistDot=on  SenseIncDot=off  SenseXDDot=off  SenseYDDot=off  SenseZDDot=off  SenseRadDDot=off  SenseAzimDDot=off  SenseDistDDot=off  SenseIncDDot=off
  cable force computation : MATLAB Function  TreatAsAtomicUnit=on
  parameter selection : Subsystem
  TO : PMIOPort  Side=Right
  FROM : PMIOPort  Port=2  Side=Right
  Fc : Outport
  wires:
  i/1 -> parameter selection/1(i)
  PS-Simulink Converter2/1 -> cable force computation/5(v)
  PS-Simulink Converter1/1 -> cable force computation/4(l)
  parameter selection/1(k) -> cable force computation/1(k)
  parameter selection/3(l0) -> Gain/1
  parameter selection/2(b) -> cable force computation/2(b)
  cable force computation/1(Fc) -> Fc/1
  Gain/1 -> cable force computation/3(l0)
  connections:
  Transform Sensor/LConn1 -- FROM/RConn1
  Transform Sensor/RConn1 -- TO/RConn1
  Transform Sensor/RConn2 -- PS-Simulink Converter1/LConn1
  Transform Sensor/RConn3 -- PS-Simulink Converter2/LConn1

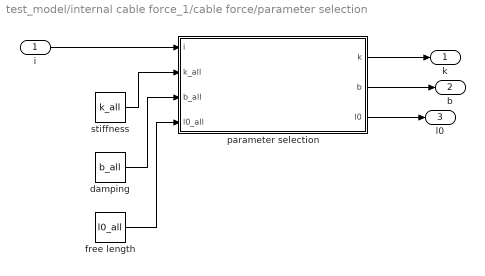
== system test_model/internal cable force_1/cable force/parameter selection ==
  i : Inport
  damping : Constant  Value=b_all
  free length : Constant  Value=l0_all
  parameter selection : MATLAB Function  TreatAsAtomicUnit=on
  stiffness : Constant  Value=k_all
  k : Outport
  b : Outport  Port=2
  l0 : Outport  Port=3
  wires:
  damping/1 -> parameter selection/3(b_all)
  stiffness/1 -> parameter selection/2(k_all)
  free length/1 -> parameter selection/4(l0_all)
  parameter selection/2(b) -> b/1
  i/1 -> parameter selection/1(i)
  parameter selection/3(l0) -> l0/1
  parameter selection/1(k) -> k/1

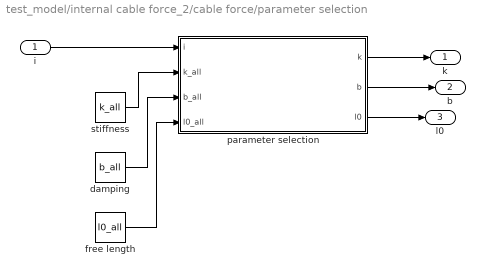
== system test_model/internal cable force_2/cable force/parameter selection ==
  i : Inport
  damping : Constant  Value=b_all
  free length : Constant  Value=l0_all
  parameter selection : MATLAB Function  TreatAsAtomicUnit=on
  stiffness : Constant  Value=k_all
  k : Outport
  b : Outport  Port=2
  l0 : Outport  Port=3
  wires:
  parameter selection/1(k) -> k/1
  parameter selection/3(l0) -> l0/1
  i/1 -> parameter selection/1(i)
  parameter selection/2(b) -> b/1
  free length/1 -> parameter selection/4(l0_all)
  stiffness/1 -> parameter selection/2(k_all)
  damping/1 -> parameter selection/3(b_all)

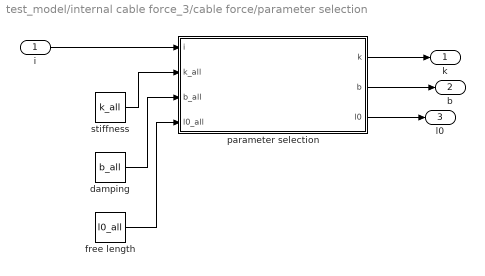
== system test_model/internal cable force_3/cable force/parameter selection ==
  i : Inport
  damping : Constant  Value=b_all
  free length : Constant  Value=l0_all
  parameter selection : MATLAB Function  TreatAsAtomicUnit=on
  stiffness : Constant  Value=k_all
  k : Outport
  b : Outport  Port=2
  l0 : Outport  Port=3
  wires:
  damping/1 -> parameter selection/3(b_all)
  stiffness/1 -> parameter selection/2(k_all)
  free length/1 -> parameter selection/4(l0_all)
  parameter selection/2(b) -> b/1
  i/1 -> parameter selection/1(i)
  parameter selection/3(l0) -> l0/1
  parameter selection/1(k) -> k/1

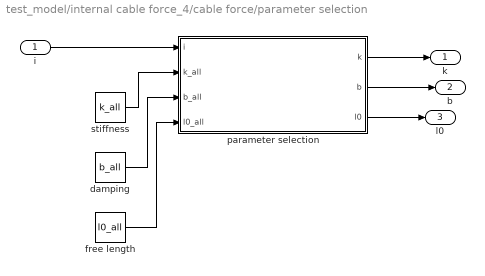
== system test_model/internal cable force_4/cable force/parameter selection ==
  i : Inport
  damping : Constant  Value=b_all
  free length : Constant  Value=l0_all
  parameter selection : MATLAB Function  TreatAsAtomicUnit=on
  stiffness : Constant  Value=k_all
  k : Outport
  b : Outport  Port=2
  l0 : Outport  Port=3
  wires:
  parameter selection/1(k) -> k/1
  parameter selection/3(l0) -> l0/1
  i/1 -> parameter selection/1(i)
  parameter selection/2(b) -> b/1
  free length/1 -> parameter selection/4(l0_all)
  stiffness/1 -> parameter selection/2(k_all)
  damping/1 -> parameter selection/3(b_all)

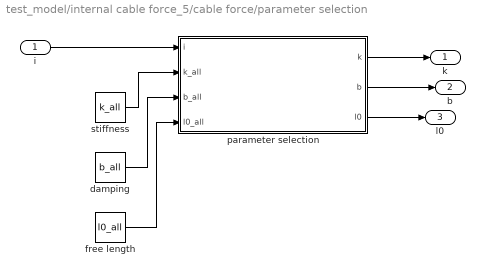
== system test_model/internal cable force_5/cable force/parameter selection ==
  i : Inport
  damping : Constant  Value=b_all
  free length : Constant  Value=l0_all
  parameter selection : MATLAB Function  TreatAsAtomicUnit=on
  stiffness : Constant  Value=k_all
  k : Outport
  b : Outport  Port=2
  l0 : Outport  Port=3
  wires:
  damping/1 -> parameter selection/3(b_all)
  stiffness/1 -> parameter selection/2(k_all)
  free length/1 -> parameter selection/4(l0_all)
  parameter selection/2(b) -> b/1
  i/1 -> parameter selection/1(i)
  parameter selection/3(l0) -> l0/1
  parameter selection/1(k) -> k/1

== system test_model/internal cable force_6/cable force/parameter selection ==
  i : Inport
  damping : Constant  Value=b_all
  free length : Constant  Value=l0_all
  parameter selection : MATLAB Function  TreatAsAtomicUnit=on
  stiffness : Constant  Value=k_all
  k : Outport
  b : Outport  Port=2
  l0 : Outport  Port=3
  wires:
  parameter selection/1(k) -> k/1
  parameter selection/3(l0) -> l0/1
  i/1 -> parameter selection/1(i)
  parameter selection/2(b) -> b/1
  free length/1 -> parameter selection/4(l0_all)
  stiffness/1 -> parameter selection/2(k_all)
  damping/1 -> parameter selection/3(b_all)

== matlab function test_model/internal cable force_5/cable force/cable force computation ==
  data: k input; Fc output; b input; l0 input; l input; v input
function Fc = cable_force(k, b,l0, l, v)

Fc=k*(l-l0) + b*v;

== matlab function test_model/internal cable force_5/cable force/parameter selection/parameter selection ==
  data: i input; k output; k_all input; b_all input; l0_all input; b output; l0 output
function [k, b, l0] = parameter_selection(i, k_all, b_all, l0_all)

k=k_all(i);
b=b_all(i);
l0=l0_all(i);

== matlab function test_model/internal cable force_1/cable force/parameter selection/parameter selection ==
  data: i input; k output; k_all input; b_all input; l0_all input; b output; l0 output
function [k, b, l0] = parameter_selection(i, k_all, b_all, l0_all)

k=k_all(i);
b=b_all(i);
l0=l0_all(i);

== matlab function test_model/internal cable force_6/cable force/cable force computation ==
  data: k input; Fc output; b input; l0 input; l input; v input
function Fc = cable_force(k, b,l0, l, v)

Fc=k*(l-l0) + b*v;

== matlab function test_model/internal cable force_6/cable force/parameter selection/parameter selection ==
  data: i input; k output; k_all input; b_all input; l0_all input; b output; l0 output
function [k, b, l0] = parameter_selection(i, k_all, b_all, l0_all)

k=k_all(i);
b=b_all(i);
l0=l0_all(i);

== matlab function test_model/internal cable force_1/cable force/cable force computation ==
  data: k input; Fc output; b input; l0 input; l input; v input
function Fc = cable_force(k, b,l0, l, v)

Fc=k*(l-l0) + b*v;

== matlab function test_model/internal cable force_2/cable force/cable force computation ==
  data: k input; Fc output; b input; l0 input; l input; v input
function Fc = cable_force(k, b,l0, l, v)

Fc=k*(l-l0) + b*v;

== matlab function test_model/internal cable force_2/cable force/parameter selection/parameter selection ==
  data: i input; k output; k_all input; b_all input; l0_all input; b output; l0 output
function [k, b, l0] = parameter_selection(i, k_all, b_all, l0_all)

k=k_all(i);
b=b_all(i);
l0=l0_all(i);

== matlab function test_model/internal cable force_3/cable force/cable force computation ==
  data: k input; Fc output; b input; l0 input; l input; v input
function Fc = cable_force(k, b,l0, l, v)

Fc=k*(l-l0) + b*v;

== matlab function test_model/internal cable force_3/cable force/parameter selection/parameter selection ==
  data: i input; k output; k_all input; b_all input; l0_all input; b output; l0 output
function [k, b, l0] = parameter_selection(i, k_all, b_all, l0_all)

k=k_all(i);
b=b_all(i);
l0=l0_all(i);

== matlab function test_model/internal cable force_4/cable force/cable force computation ==
  data: k input; Fc output; b input; l0 input; l input; v input
function Fc = cable_force(k, b,l0, l, v)

Fc=k*(l-l0) + b*v;

== matlab function test_model/internal cable force_4/cable force/parameter selection/parameter selection ==
  data: i input; k output; k_all input; b_all input; l0_all input; b output; l0 output
function [k, b, l0] = parameter_selection(i, k_all, b_all, l0_all)

k=k_all(i);
b=b_all(i);
l0=l0_all(i);
